simulink model "Masseschwinger_Konstant"  (R2026a)
settings: Solver=ode3  StopTime=30  FixedStep=0.0001
settings Model: Creator=alfa  LastModifiedBy=alfa

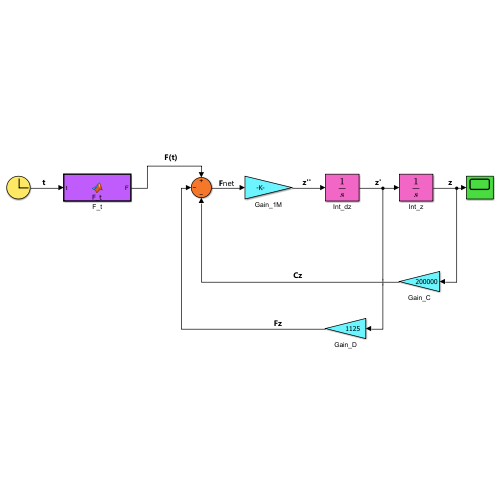
[thumbnail: Simulink's stored preview of the top-level diagram]
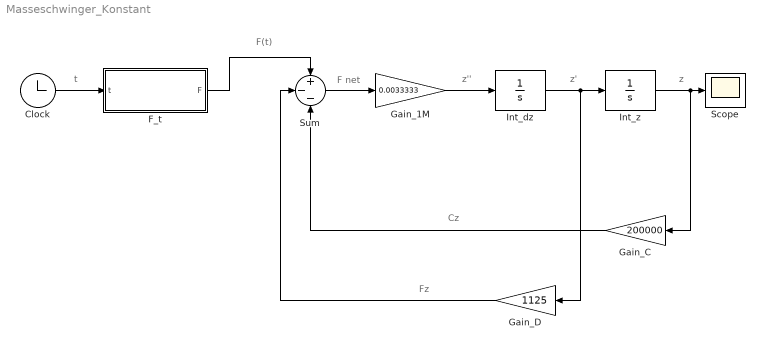
== system Masseschwinger_Konstant ==
  note: t
  note: F net
  note: F(t)
  note: Fz
  note: Cz
  note: z''
  note: z'
  note: z
  Clock : Clock
  F_t : MATLAB Function  TreatAsAtomicUnit=on
  Gain_1M : Gain  Gain=0.0033333
  Gain_C : Gain  Gain=200000
  Gain_D : Gain  Gain=1125
  Int_dz : Integrator
  Int_z : Integrator
  Scope : Scope
      settings: ActiveDisplayYMinimum=-0.001018976276959577  ActiveDisplayYMaximum=0.0091707864926361959
  Sum : Sum  Inputs=+--
  wires:
  F_t/1(F) -> Sum/1
  Sum/1 -> Gain_1M/1
  Gain_1M/1 -> Int_dz/1
  Int_dz/1 -> Int_z/1, Gain_D/1
  Int_z/1 -> Scope/1, Gain_C/1
  Clock/1 -> F_t/1(t)
  Gain_C/1 -> Sum/3
  Gain_D/1 -> Sum/2

== matlab function Masseschwinger_Konstant/F_t ==
  data: t input; F output
function F = F_t(t)
  H = 1111.0;
  omega = 0.90;
  F = 0.5*H*(t>=3) + H*((t>=1)-(t>=3))*sin(omega*t);
end
